simulink model "Mass_spring_damping_control_simulation"  (R2015b)
settings: Solver=VariableStepAuto  StartTime=0.0  StopTime=300  RelTol=1e-3
settings Model: Creator=99155071  LastModifiedBy=99155071

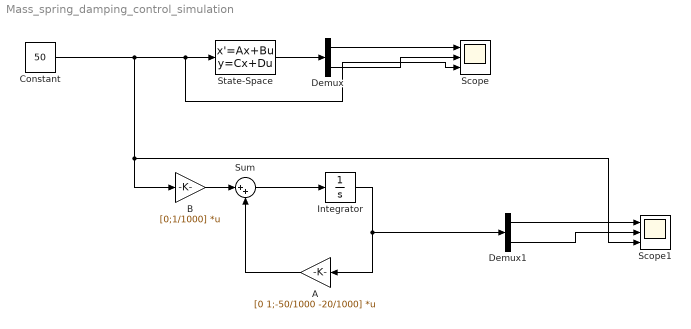
== system Mass_spring_damping_control_simulation ==
  A : Gain  Gain=[0 1;-50/1000 -20/1000]  Multiplication=Matrix(K*u)
  B : Gain  Gain=[0;1/1000]  Multiplication=Matrix(K*u)
  Constant : Constant  Value=50
  Demux : Demux  Outputs=2
  Demux1 : Demux  Outputs=2
  Integrator : Integrator
  Scope : Scope  NumInputPorts=3
  Scope1 : Scope  NumInputPorts=3
  State-Space : StateSpace  A=[0 1;-50/1000 -20/1000]  B=[0;1/1000]  C=[1 0; 0 1]  D=[0;0]  X0=[0; 0]
  Sum : Sum  Inputs=|++
  wires:
  Constant/1 -> B/1, Scope1/3, Scope/3, State-Space/1
  Demux/1 -> Scope/1
  Demux/2 -> Scope/2
  State-Space/1 -> Demux/1
  B/1 -> Sum/1
  A/1 -> Sum/2
  Sum/1 -> Integrator/1
  Integrator/1 -> Demux1/1, A/1
  Demux1/1 -> Scope1/1
  Demux1/2 -> Scope1/2
